simulink model "Older_model_ contains_ACC"  (R2023b)
settings: Solver=VariableStepAuto  StartTime=0.0  StopTime=30  MaxStep=1e-2  RelTol=1e-3  AbsTol=1e-3
values from neighbouring files (symbols this model uses):
  b = 1.6    [a2024_v2x_matlab_6veh.m]
  m = 2000    [a2024_v2x_matlab_6veh.m]
  mEgo = 1500    [a2024_v2x_matlab_6veh.m]
  sampleTime = 0.1    [a2024_v2x_matlab_6veh.m]    (also in v2x_matlab.m; v2x_matlabV2.m; v2x_matlab_6veh.m; v2x_matlab_R.m)
  t_gap = 1.4    [a2024_v2x_matlab_6veh.m]
  waypoints = [egoWP(:,2) egoWP(:,1), zeroforwp]    [a2024_v2x_matlab_6veh.m]    (also in misc.m = data.data.ActorSpecifications(1,1).Waypoints(:,[1,2]); v2x_matlab.m = data.data.ActorSpecifications(1,1).Waypoints(:,[1,2]); v2x_matlabV2.m = [5 -1.6 0; v2x_matlab_R.m = [5 -1.6 0)
  ZeroActors = struct(     'ActorID',0,     'Position', [1000 1000 1000],      'Velocity', [0 0 0],      'Roll', 0,      'Pitch', 0,      'Yaw', 0,      'AngularVelocity', [0 0 0])    [v2x_matlabV2.m]    (also in v2x_matlab_R.m)
undefined symbols (not defined in the file or in its folder): doppler, driving, n, PredictionHorizon, Ts
libraries: simulink x13, simulink_extras x12, commofdm x10, commdigbbndam3 x10, commchan3 x3, drivingscenarioandsensors x3, mpcadaslib x2, commsink2 x2, vehdynlibdriver x1, dspmathops x1, autolibshared x1
(part 1 of 3)
settings Model: DataDictionary=V2X.sldd  Creator=Fauszt Gábor  LastModifiedBy=Fauszt Gábor

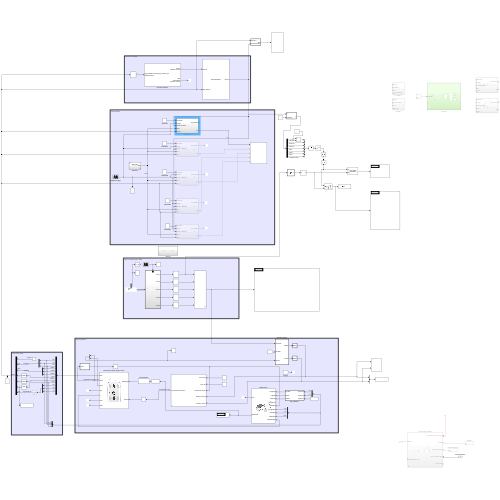
[thumbnail: Simulink's stored preview of the top-level diagram]
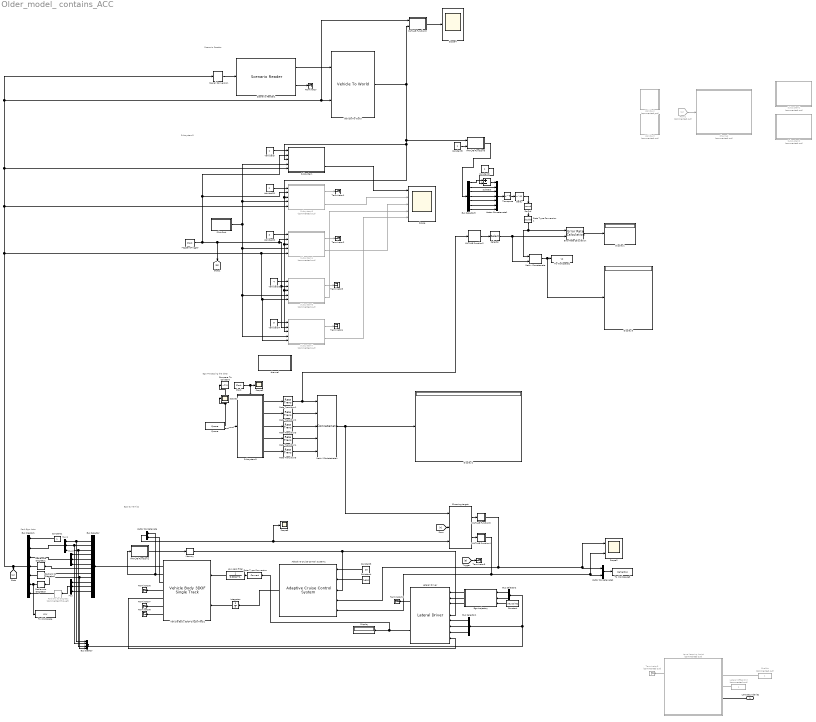
== system Older_model_ contains_ACC ==
  note: Ego Dynamics
  note: Ego Processing the data
  note: Subsystem3
  note: Scenario Reader
  note: Pack Ego Actor
  Lane Boundaries : Inport
  Adaptive Cruise Control System1 : mpcadaslib/Adaptive Cruise Control System  EgoModel=tf(1,[0.5,1,0])  InitialEgoVelocity=20  DefaultSpacing=0  MaxVelocity=20  MinAcceleration=-2  amin_ext=off  MaxAcceleration=4  amax_ext=off  Ts=0.01  PredictionHorizon=3  ControllerBehavior=0.950  suboptimal=off  maxiter=10  datatypeopt=double  optmode=off  trackmode=off
      settings: LibrarySourceBlock=mpclib/Automated Driving/Adaptive Cruise Control System
  Bus Creator : BusCreator  Inputs=4
  Bus Creator1 : BusCreator  Inputs=7  OutDataTypeStr=Bus: Actors
      settings: InheritFromInputs=off
  Bus Selector : BusSelector  OutputSignals=InertFrm.Cg.Disp.X,InertFrm.Cg.Disp.Y,InertFrm.Cg.Disp.Z,InertFrm.Cg.Vel.Xdot,InertFrm.Cg.Vel.Ydot,InertFrm.Cg.Vel.Zdot,InertFrm.Cg.Ang.phi,InertFrm.Cg.Ang.theta,InertFrm.Cg.Ang.psi,BdyFrm.Cg.AngVel.p,BdyFrm.Cg.AngVel.q,BdyFrm.Cg.AngVel.r
  Bus Selector1 : BusSelector  OutputSignals=X,Y,psi
  Bus Selector2 : BusSelector  OutputSignals=X,Y
  Bus Selector3 : BusSelector  OutputSignals=ActorID,Position,Velocity,Roll,Pitch,Yaw,AngularVelocity
  Channel : Subsystem  Commented=on
  "Choosing target " : MATLAB Function  TreatAsAtomicUnit=on
  Clock : simulink_extras/Flip Flops/Clock  period=0.01
  Compare To Constant : simulink/Logic and Bit Operations/Compare To Constant  relop=~=  const=0  OutDataTypeStr=uint8
  Constant : Constant  Value=waypoints
  Constant1 : Constant  SampleTime=-1
  Constant2 : Constant
  Constant3 : Constant  Value=20  VectorParams1D=off  SampleTime=sampleTime
  Constant4 : Constant  Value=t_gap  VectorParams1D=off  SampleTime=sampleTime
  Constant5 : Constant
  Data Type Conversion : DataTypeConversion  SaturateOnIntegerOverflow=off  RndMeth=Floor
  Data Type Conversion1 : DataTypeConversion  OutDataTypeStr=double  SaturateOnIntegerOverflow=off  RndMeth=Floor
  Delay : Delay  DelayLength=11
  Display{,1..3} (4 alike) : Display
  Ego trajectory : MATLAB Function  TreatAsAtomicUnit=on
  Enable : Constant  Commented=on
  Error Rate Calculation : commsink2/Error Rate Calculation  N=0  st_delay=0  cp_mode=Entire frame  subframe=[]  PMode=Port  WsName=ErrorVec  RsMode2=off  stop=off  numErr=100  maxBits=1e6
      settings: LibrarySourceBlock=|
      | commhdlsink/Error Rate
      | Calculation
  From : From
  From1 : From  Commented=on
  Goto : Goto
  Integrator : Integrator
  Lane Keeping Assist : Subsystem  Commented=on
  Lateral Driver : vehdynlibdriver/Lateral Driver  extSteerOvr=off  extSteerHld=off  extSteerZero=off  steerOut=off  cntrlTypeLat=Stanley  coordMode=SAE J670 (Z-down)  angUnits=rad  tau=0.1  L=3  vecPose=off  dynamMode=on  PositionGainF=2.5  PositionGainR=2.5  YawRateGain=.2  DelayGain=.2  a=a  b=b  m=mEgo  Cy_f=Cy_f  Cy_r=70933  I=4013  Ksteer=18  theta=45*pi/180  aMode=2
  Lateral Offset [m] : Constant  Commented=on
  Low pass filter : TransferFcn  Denominator=[0.001 1]
  MATLAB Function1 : MATLAB Function  TreatAsAtomicUnit=on
  MATLAB Function2 : MATLAB Function  TreatAsAtomicUnit=on
  MATLAB Function3 : MATLAB Function  TreatAsAtomicUnit=on
  MATLAB Function4 : MATLAB Function  TreatAsAtomicUnit=on
  MATLAB Function5 : MATLAB Function  TreatAsAtomicUnit=on
  MATLAB Function6 : MATLAB Function  TreatAsAtomicUnit=on
  Matrix Concatenate : Concatenate  Mode=Multidimensional array  ConcatenateDimension=2
  Matrix Concatenate1 : Concatenate  NumInputs=5  Mode=Multidimensional array  ConcatenateDimension=2
  Memory : Memory  InitialCondition=1
  MsgSendTrigger : simulink_extras/Flip Flops/Clock  period=0.1
  Mux : Mux  Inputs=3
  Mux1 : Mux  Inputs=3
  Mux2 : Mux  Inputs=3
  Pilot Port : Subsystem  ReferencedSubsystem=Pilot_Port
  Queue : Queue  OutputPortMessageModes=n,m  Capacity=5  EntityArrivalSource=Multicast  MulticastTag=B  NumberEntitiesInBlock=on
      settings: OutputPortMap=o1,o5
  Radians to Degrees : simulink_extras/Transformations/Radians to Degrees  Commented=through
  Radians to Degrees1 : simulink_extras/Transformations/Radians to Degrees
  Radians to Degrees2 : simulink_extras/Transformations/Radians to Degrees
  Radians to Degrees3 : simulink_extras/Transformations/Radians to Degrees
  Rate Transition{1..5} (5 alike) : RateTransition  OutPortSampleTime=sampleTime/10
  Round : Rounding  Operator=round
  Scenario Reader1 : drivingscenarioandsensors/Scenario Reader  ScenarioSource=From file  ScenarioFileName=C:\Users\Fauszt Gábor\OneDrive - Budapesti Műszaki és Gazdaságtudományi Egyetem\Projekt - Diplomamunka\MODELL\driving_scenario_4V.mat  ScenarioVariableName=scenario  OutputCoordinateSystem=Vehicle coordinates  EgoVehicleSource=Input port  EgoVehicleActorID=1  OrientVehiclesOnRoad=off  OutputEgoVehiclePose=on  OutputEgoVehicleState=off  SampleTime=sampleTime  LaneBoundaryOutput=All lane boundaries  LaneBoundaryDistance=0:0.5:9.5  LaneBoundaryLocation=Center of lane markings  BusNameSource=Auto  BusName=ActorsAll  BusNumActorsSource=Scenario  BusNumActors=100  BusName2Source=Auto  BusName2=BusLaneBoundaries  BusNumLaneBoundariesSource=Scenario  BusNumLaneBoundaries=10  BusName3Source=Auto  BusName3=BusEgoActor  BusName4Source=Auto  BusName4=BusEgoState  ShowCoordinateLabels=on  SimulateUsing=Interpreted execution
  Scope : Scope  NumInputPorts=5
  Scope{1,3..5} (4 alike) : Scope
  Scope2 : Scope  NumInputPorts=2
  Selector : Selector  InputPortWidth=15  IndexOptions=Starting index (dialog)  Indices=3  OutputSizes=13
  Signal Conversion : SignalConversion  ConversionOutput=Nonvirtual bus  OverrideOpt=off
  Subsystem : Subsystem
  Subsystem1 : Subsystem  Commented=on
  Subsystem2 : Subsystem  Commented=on
  Subsystem3 : Subsystem
  Subsystem4 : Subsystem  Commented=on
  Subsystem5 : Subsystem  Commented=on
  Subsystem6 : Subsystem  Commented=on
  Subsystem7 : Subsystem  Commented=on
  Subtract : Sum  Inputs=+-
  Terminator{,1..8,10} (10 alike) : Terminator
  Terminator9 : Terminator  Commented=on
  To Workspace : ToWorkspace  VariableName=yaw  SampleTime=-1
  To Workspace1 : ToWorkspace  VariableName=V2  SampleTime=-1
  To Workspace3 : ToWorkspace  VariableName=RelVelPos  SampleTime=-1
  Transpose : Math  Operator=transpose
  Vector Concatenate : Concatenate
  Vector Concatenate1 : Concatenate  NumInputs=7
  Vector Concatenate2 : Concatenate
  Vehicle 2 : Subsystem  Commented=on
  Vehicle 3 : Subsystem  Commented=on
  Vehicle Body 3DOF Single Track1 : autolibshared/Vehicle Body 3DOF Single Track  trackMode=Single (bicycle)  inputMode=External longitudinal velocity  frontSteerMode=on  rearSteerMode=off  windMode=off  muMode=off  extFMode=off  extMMode=off  htchFMode=off  htchMMode=off  extXo=off  extpsio=off  extxdoto=off  extro=off  extYo=off  extTamb=off  extydoto=off  aMode=2  NF=nrWheelsFr  NR=nrWheelsRe  m=mEgo  a=a  b=b  h=h  dh=1  hh=0.2  X_o=waypoints(1,1)  xdot_o=0  CalphaMode=off  sigmaMode=on  d=0  hl=0  w=[1.4,1.4]  Cy_f=Cy_f  Cy_r=Cy_r  sigma_f=sigma_f  sigma_r=sigma_r  alpha_f_brk=[-.1 .1]  Cy_f_data=[-9e3 9e3]  alpha_r_brk=[-.1 .1]  Cy_r_data=[-9e3 9e3]  Y_o=waypoints(1,2)  ydot_o=0  Izz=Izz  psi_o=deg2rad(waypoints(1,3))  r_o=deg2rad(waypoints(1,3))  Af=2  Cd=.3  Cl=.1  Cpm=.1  beta_w=[0 0.01:0.01:0.3]  Cs=[0 0.01:0.01:0.3]  Cym=[0 1e-6:0.01:0.3]  Pabs=101325  Tair=273  g=9.81  mu=1  xdot_tol=.01  Fznom=5000  Fxtire_sat=7e4  Fytire_sat=7e4  longOff=0  latOff=0  vertOff=0  wrapAng=off
  Vehicle To World : drivingscenarioandsensors/Vehicle To World  BusNameSource=Auto  BusName=ActorsaAll  SimulateUsing=Interpreted execution
  VehicleID : Constant
  VehicleID1 : Constant  Value=2
  VehicleID2 : Constant  Value=3
  VehicleID3 : Constant  Value=4
  VehicleID4 : Constant  Value=5
  channel : Subsystem
  wires:
  From1/1 -> Channel/1(EgoData)
  Lateral Offset [m]/1 -> Lane Keeping Assist/3(Lane Assist Offset)
  Lane Keeping Assist/1(Status) -> Terminator9/1
  Lane Boundaries/1 -> Lane Keeping Assist/4(lane boundaries Bus)
  Enable/1 -> Lane Keeping Assist/2(Enable)
  ? -> Lane Keeping Assist/1(Longitudinal velocity of ego)
  Scenario Reader1/1 -> Vehicle To World/1
  Bus Selector/6 -> Mux2/3  "<Zdot>"
  Bus Selector/5 -> Mux2/2  "<Ydot>"
  Constant1/1 -> Bus Creator1/1  "ActorID"
  Bus Selector/4 -> Mux2/1  "<Xdot>"
  Mux1/1 -> Bus Creator1/2  "Position"
  Bus Creator1/1 -> MATLAB Function3/1(EgoActor), Vehicle To World/2, Signal Conversion/1, Subsystem/5(Actors), Subsystem5/5(Actors), Subsystem7/5(Actors), Subsystem6/5(Actors), Subsystem4/5(Actors), Goto/1  "Actors"
  Bus Selector/7 -> Radians to Degrees1/1  "<phi>"
  Bus Selector/1 -> Bus Creator/1, Mux1/1  "<X>"
  Radians to Degrees/1 -> Bus Creator1/7  "AngularVelocity"
  Bus Selector/2 -> Bus Creator/2, Mux1/2  "<Y>"
  Bus Selector/10 -> Mux/1  "<p>"
  Bus Selector/8 -> Radians to Degrees2/1  "<theta>"
  Bus Selector/3 -> Mux1/3, Bus Creator/3  "<Z>"
  Mux/1 -> Radians to Degrees/1
  Mux2/1 -> Bus Creator1/3  "Velocity"
  Bus Selector/9 -> Radians to Degrees3/1, Bus Creator/4  "<psi>"
  Bus Selector/12 -> Mux/3  "<r>"
  Bus Selector/11 -> Mux/2  "<q>"
  Vehicle Body 3DOF Single Track1/1 -> Bus Selector/1
  MsgSendTrigger/1 -> Subsystem7/2(Trigger), Subsystem6/2(Trigger), Subsystem4/2(Trigger), [B], Subsystem5/2(Trigger), Subsystem/2(Trigger)
  Signal Conversion/1 -> Scenario Reader1/1
  Scenario Reader1/2 -> Terminator/1
  Radians to Degrees1/1 -> Bus Creator1/4
  Radians to Degrees2/1 -> Bus Creator1/5
  Radians to Degrees3/1 -> To Workspace/1, Bus Creator1/6
  VehicleID1/1 -> Subsystem5/1(VehicleID)
  VehicleID/1 -> Subsystem/1(VehicleID)
  Subsystem4/2(V3) -> Scope/3  "V3"
  VehicleID2/1 -> Subsystem4/1(VehicleID)
  Subsystem4/1(VehicleData) -> Terminator2/1
  Subsystem5/2(V2) -> Scope/2  "V2"
  Subsystem/2(V1) -> Scope/1  "V1"
  Vehicle To World/1 -> MATLAB Function3/2(busActors3Test1), Subsystem7/3(busActors3Test1), Subsystem6/3(busActors3Test1), Subsystem4/3(busActors3Test1), Subsystem5/3(busActors3Test1), Subsystem/3(busActors3Test1), MATLAB Function6/1(u)
  Pilot Port/1 -> Subsystem7/4(Pilot), Subsystem6/4(Pilot), Subsystem4/4(Pilot), Subsystem5/4(Pilot), Subsystem/4(Pilot)  "Pilot"
  Subsystem5/1(VehicleData) -> Terminator1/1
  [B] -> Terminator5/1
  Vector Concatenate/1 -> Scope5/1, "Choosing target "/3(EgoVel)
  Subsystem3/2(Actor2) -> Rate Transition2/1
  Matrix Concatenate1/1 -> Display2/1, "Choosing target "/1(ActorsMX)
  Subsystem3/1(Actor1) -> Rate Transition1/1
  Subsystem3/3(Actor3) -> Rate Transition3/1
  From/1 -> "Choosing target "/2(EgoData)
  Subsystem3/4(Actor4) -> Rate Transition4/1
  Queue/1 -> Compare To Constant/1, Scope1/1
  Queue/2 -> Subsystem3/1(In1)
  "Choosing target "/1(RelDist) -> MATLAB Function5/1(u)
  Bus Creator/1 -> Bus Selector2/1, Bus Selector1/1
  Memory/1 -> Lateral Driver/5, Adaptive Cruise Control System1/3
  Vehicle Body 3DOF Single Track1/2 -> Vector Concatenate/1, MATLAB Function1/1(xdotin)  "Longitudinal velocity of ego"
  Lateral Driver/1 -> Terminator10/1
  Vehicle Body 3DOF Single Track1/3 -> Vector Concatenate/2
  Data Type Conversion/1 -> Low pass filter/1
  Ego trajectory/2(LatRef) -> Lateral Driver/2
  Vehicle Body 3DOF Single Track1/5 -> Lateral Driver/9  "r"
  Bus Selector2/2 -> Ego trajectory/2(EgoFdbY)  "<Y>"
  Vehicle Body 3DOF Single Track1/6 -> Terminator7/1
  "Choosing target "/2(RelVel) -> MATLAB Function4/1(u)
  Constant/1 -> Ego trajectory/3(waypoints)
  Bus Selector1/3 -> Lateral Driver/8  "<psi>"
  Bus Selector1/1 -> Lateral Driver/6  "<X>"
  Vehicle Body 3DOF Single Track1/4 -> Terminator6/1
  Ego trajectory/1(LongRef) -> Lateral Driver/1
  Integrator/1 -> Vehicle Body 3DOF Single Track1/2
  Ego trajectory/3(YawRef) -> Lateral Driver/3
  MATLAB Function1/1(y) -> Memory/1
  Constant3/1 -> Adaptive Cruise Control System1/1
  Vehicle Body 3DOF Single Track1/7 -> Terminator8/1
  Constant4/1 -> Adaptive Cruise Control System1/2
  Low pass filter/1 -> Vehicle Body 3DOF Single Track1/1
  Bus Selector2/1 -> Ego trajectory/1(EgoFdbX)  "<X>"
  Adaptive Cruise Control System1/1 -> Integrator/1  "Acceleration of ego"
  Bus Selector1/2 -> Lateral Driver/7  "<Y>"
  Lateral Driver/2 -> Data Type Conversion/1, Display/1
  Vector Concatenate1/1 -> Transpose/1
  Bus Selector3/2 -> Vector Concatenate1/2  "<Position>"
  Bus Selector3/3 -> Vector Concatenate1/3  "<Velocity>"
  Bus Selector3/4 -> Vector Concatenate1/4  "<Roll>"
  Bus Selector3/5 -> Vector Concatenate1/5  "<Pitch>"
  Bus Selector3/6 -> Vector Concatenate1/6  "<Yaw>"
  Bus Selector3/7 -> Vector Concatenate1/7  "<AngularVelocity>"
  Selector/1 -> Matrix Concatenate/2, Error Rate Calculation/2
  Transpose/1 -> Delay/1
  MATLAB Function2/1(y) -> Selector/1
  Data Type Conversion1/1 -> Error Rate Calculation/1, Matrix Concatenate/1
  Error Rate Calculation/1 -> Display1/1
  MATLAB Function3/1(Dist) -> Scope4/1
  Matrix Concatenate/1 -> Display3/1, To Workspace1/1
  Round/1 -> Data Type Conversion1/1
  Vector Concatenate2/1 -> To Workspace3/1
  MATLAB Function4/1(RelVel) -> Adaptive Cruise Control System1/5, Scope2/2, Vector Concatenate2/2
  MATLAB Function5/1(RelDist) -> Adaptive Cruise Control System1/4, Vector Concatenate2/1, Scope2/1
  Delay/1 -> Round/1
  Clock/1 -> Scope3/1, Subsystem3/Enable
  Rate Transition3/1 -> Matrix Concatenate1/3
  Rate Transition2/1 -> Matrix Concatenate1/2
  Rate Transition1/1 -> MATLAB Function2/1(u), Matrix Concatenate1/1
  Rate Transition4/1 -> Matrix Concatenate1/4
  MATLAB Function6/1(y) -> Bus Selector3/1
  VehicleID3/1 -> Subsystem6/1(VehicleID)
  VehicleID4/1 -> Subsystem7/1(VehicleID)
  Subsystem6/1(VehicleData) -> Terminator3/1
  Subsystem7/1(VehicleData) -> Terminator4/1
  Subsystem3/5(Actor5) -> Rate Transition5/1
  Rate Transition5/1 -> Matrix Concatenate1/5
  Subsystem6/2(V4) -> Scope/4  "V4"
  Subsystem7/2(V5) -> Scope/5  "V3"
  Bus Selector3/1 -> Subtract/1  "<ActorID>"
  Subtract/1 -> Vector Concatenate1/1
  Constant2/1 -> Subtract/2
  Constant5/1 -> MATLAB Function6/2(vehicleID)

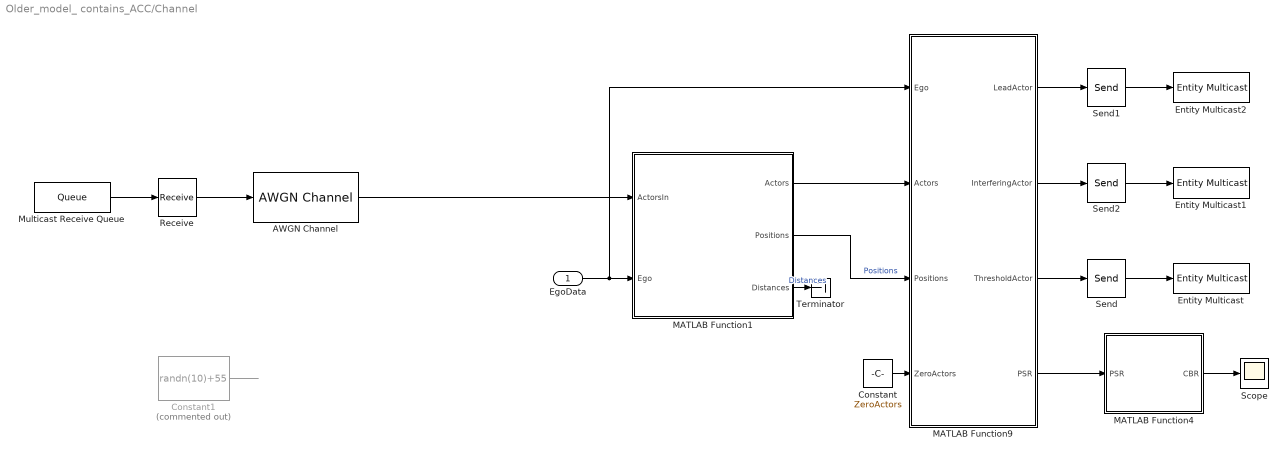
== system Older_model_ contains_ACC/Channel ==
  EgoData : Inport
  AWGN Channel : commchan3/AWGN Channel  LegacyMode=off  NoiseMethod="Signal to noise ratio  (SNR)"  noiseMode="Signal to noise ratio  (SNR)"  EbNo=10  EsNo=10  SNR=60  BitsPerSymbol=1  SignalPower=1  SamplesPerSymbol=1  SymbolPeriod=1  VarianceSource=Parameter  Variance=1  RandomStream=Global stream  Seed=67  SimulateUsing=Interpreted execution
  Constant : Constant  Value=ZeroActors  OutDataTypeStr=Bus: Actors  SampleTime=sampleTime
  Constant1 : Constant  Commented=on  Value=randn(10)+55  SampleTime=sampleTime
  Entity Multicast : EntityMulticast  InputPortMessageModes=m  MulticastTag=B
  Entity Multicast1 : EntityMulticast  InputPortMessageModes=m  MulticastTag=B
  Entity Multicast2 : EntityMulticast  InputPortMessageModes=m  MulticastTag=B
  MATLAB Function1 : MATLAB Function  TreatAsAtomicUnit=on
  MATLAB Function4 : MATLAB Function  TreatAsAtomicUnit=on
  MATLAB Function9 : MATLAB Function  TreatAsAtomicUnit=on
  Multicast Receive Queue : Queue  OutputPortMessageModes=m  EntityArrivalSource=Multicast
  Receive : Receive  InputPortMessageModes=m  UseInternalQueue=off  QueueOverwriting=on  QueueLength=1  QueueType=LIFO
  Scope : Scope
  Send : Send  OutputPortMessageModes=m
  Send1 : Send  OutputPortMessageModes=m
  Send2 : Send  OutputPortMessageModes=m
  Terminator : Terminator
  wires:
  Multicast Receive Queue/1 -> Receive/1
  AWGN Channel/1 -> MATLAB Function1/1(ActorsIn)
  Receive/1 -> AWGN Channel/1
  MATLAB Function1/1(Actors) -> MATLAB Function9/2(Actors)
  MATLAB Function1/2(Positions) -> MATLAB Function9/3(Positions)  "Positions"
  Constant/1 -> MATLAB Function9/4(ZeroActors)
  MATLAB Function9/4(PSR) -> MATLAB Function4/1(PSR)
  MATLAB Function9/3(ThresholdActor) -> Send/1
  MATLAB Function9/2(InterferingActor) -> Send2/1
  MATLAB Function9/1(LeadActor) -> Send1/1
  EgoData/1 -> MATLAB Function9/1(Ego), MATLAB Function1/2(Ego)
  Constant1/1 -> ?
  MATLAB Function1/3(Distances) -> Terminator/1  "Distances"
  MATLAB Function4/1(CBR) -> Scope/1
  Send1/1 -> Entity Multicast2/1
  Send2/1 -> Entity Multicast1/1
  Send/1 -> Entity Multicast/1

== system Older_model_ contains_ACC/Lane Keeping Assist ==
  Longitudinal velocity of ego : Inport
  Enable : Inport  Port=2
  Lane Assist Offset : Inport  Port=3
  lane boundaries Bus : Inport  Port=4
  Driver Steer : Inport  Port=5
  Abs : Abs  SaturateOnIntegerOverflow=off
  Estimate lane center : Subsystem
  Lane Keeping Assist System : mpcadaslib/Lane Keeping Assist System  ModelType=Use vehicle parameters  VehicleMass=mEgo  VehicleYawInertia=2875  LengthToFront=a  LengthToRear=b  FrontTireStiffness=Cy_f  RearTireStiffness=Cy_r  EgoModelMatrixA=[-4.4021 ,-12.4603;1.3913,-5.1868]  EgoModelMatrixB=[24.1270;15.8609]  EgoModelMatrixC=[1,0;0,1]  InitialLongVel=16  TransportLag=0  MinSteering=-0.5  umin_ext=off  MaxSteering=0.5  umax_ext=off  Ts=0.1  PredictionHorizon=5  ControllerBehavior=0.100  suboptimal=off  maxiter=10  datatypeopt=double  optmode=off  trackmode=off
      link override Longitudinal velocity must be positive: stopWhenAssertionFail=on
      settings: LibrarySourceBlock=mpclib/Automated Driving/Lane Keeping Assist System
  Pack to Custom Sensor Data Format : Subsystem
  Subsystem : Subsystem
  Subsystem2 : Subsystem
  Vision Detection Generator : drivingscenarioandsensors/Vision Detection Generator  SensorIndex=1  DetectorOutput=Lanes only  UpdateInterval=0.1  LaneUpdateInterval=0.1  SensorLocation=[ 1.9, 0 ]  Height=1.1  Yaw=0  Pitch=1  Roll=0  BusNameSource=Auto  BusName=BusObjectDetections  BusName2Source=Auto  BusName2=BusLaneDetections  MaxNumDetectionsSource=Property  MaxNumDetections=50  MaxNumLanesSource=Property  MaxNumLanes=30  DetectionCoordinates=Ego Cartesian  SimulateUsing=Interpreted execution  MaxRange=10  BoundingBoxAccuracy=5  ProcessNoiseIntensity=5  MaxSpeed=100  MaxAllowedOcclusion=0.5  MinObjectImageSize=[ 15, 15 ]  DetectionProbability=0.9  FalsePositivesPerImage=0.1  MinLaneImageSize=[ 20, 3 ]  LaneBoundaryAccuracy=3  HasNoise=on  InitialSeedSource=Repeatable  InitialSeed=0  UsedSeed=driving.internal.SimulinkUtilities.seedManager(gcb)  ActorProfilesSource=From Scenario Reader block  ActorProfilesParameters=driving.internal.ActorProfilesParameters  ActorProfilesExpression=struct( 'ClassID', 0, 'Length', 4.7, 'Width', 1.8, 'Height', 1.4, 'OriginOffset', [ -1.35, 0, 0 ] )  Intrinsics=driving.internal.cameraIntrinsics('FocalLength',[1, 1 ])
  Status : Outport
  SteeringAngle in rad : Outport  Port=2
  wires:
  Subsystem/1(Departure Detected) -> Subsystem2/2(Set)
  Estimate lane center/2(Lateral Offset) -> Lane Keeping Assist System/3
  Enable/1 -> Subsystem2/1(Enable)
  Pack to Custom Sensor Data Format/1(lanes) -> Subsystem/2(Lane Sensor data), Estimate lane center/2(Lane Boundaries)
  Estimate lane center/1(Previewed Curvature) -> Lane Keeping Assist System/1
  Estimate lane center/3(Heading Angle) -> Lane Keeping Assist System/4
  lane boundaries Bus/1 -> Vision Detection Generator/1
  Vision Detection Generator/1 -> Pack to Custom Sensor Data Format/1(lane Detections)
  Lane Assist Offset/1 -> Subsystem/1(Lane Assist Offset)
  Driver Steer/1 -> Subsystem2/4(Driver Steer)
  Subsystem2/1(Status) -> Status/1
  Longitudinal velocity of ego/1 -> Abs/1, Estimate lane center/1(Longitudinal velocity of ego)
  Abs/1 -> Lane Keeping Assist System/2
  Subsystem2/2(SteeringAngle in rad) -> SteeringAngle in rad/1
  Lane Keeping Assist System/1 -> Subsystem2/3(Assisted Steer)  "Assisted Steer"

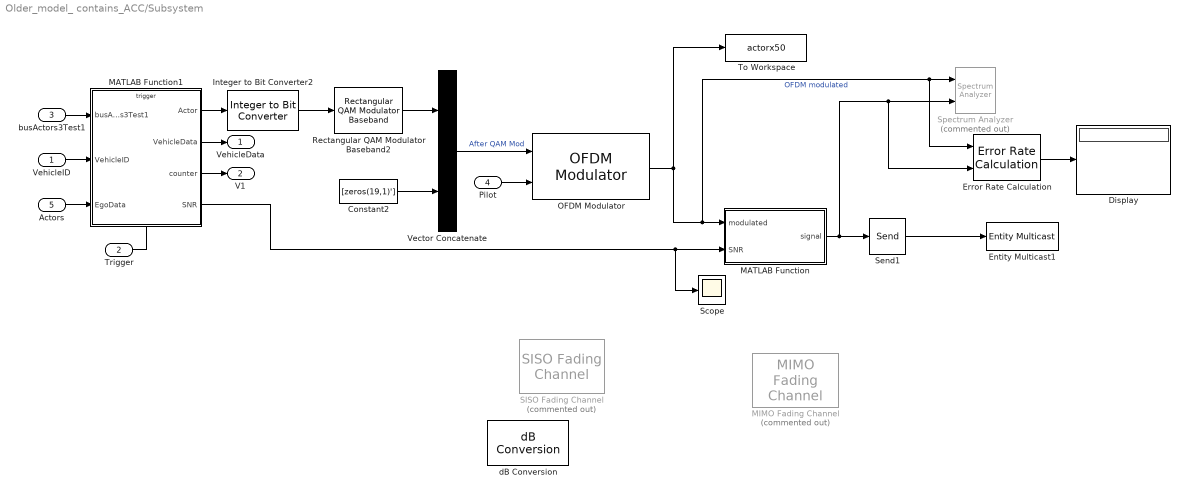
== system Older_model_ contains_ACC/Subsystem ==
  VehicleID : Inport
  Trigger : Inport  Port=2
  busActors3Test1 : Inport  Port=3
  Pilot : Inport  Port=4
  Actors : Inport  Port=5
  Constant2 : Constant  Value=[zeros(19,1)']  SampleTime=-1
  Display : Display
  Entity Multicast1 : EntityMulticast  InputPortMessageModes=m
  Error Rate Calculation : commsink2/Error Rate Calculation  N=0  st_delay=0  cp_mode=Entire frame  subframe=[]  PMode=Port  WsName=ErrorVec  RsMode2=off  stop=off  numErr=100  maxBits=1e6
      settings: LibrarySourceBlock=|
      | commhdlsink/Error Rate
      | Calculation
  Integer to Bit Converter2 : simulink/Logic and Bit Operations/Integer to Bit Converter  nbits=16  signedInputValues=Signed  bitOrder=MSB first  outDtype=boolean
  MATLAB Function : MATLAB Function  TreatAsAtomicUnit=on
  MATLAB Function1 : MATLAB Function  TreatAsAtomicUnit=on
  MIMO Fading Channel : commchan3/MIMO Fading Channel  Commented=on  InheritSampleRate=on  SampleRate=1  PathDelays=0  AveragePathGains=0  NormalizePathGains=on  FadingDistribution=Rayleigh  KFactor=3  DirectPathDopplerShift=0  DirectPathInitialPhase=0  MaximumDopplerShift=0.001  DopplerSpectrum=doppler('Jakes')  SpatialCorrelationSpecification=None  SpatialCorrelationMatrix=[1 0 0 0; 0 1 0 0; 0 0 1 0; 0 0 0 1]  NumTransmitAntennas=1  NumReceiveAntennas=1  TransmitCorrelationMatrix=[1 0; 0 1]  ReceiveCorrelationMatrix=[1 0; 0 1]  AntennaSelection=Off  NormalizeChannelOutputs=on  PathGainsOutputPort=off  SimulateUsing=Interpreted execution  FadingTechnique=Filtered Gaussian noise  NumSinusoids=48  InitialTimeSource=Property  InitialTime=0  RandomStream=mt19937ar with seed  Seed=73  Visualization=Off  AntennaPairsToDisplay=[ 1, 1 ]  PathsForDopplerDisplay=1  SamplesToDisplay=25%
  OFDM Modulator : commofdm/OFDM Modulator  StatePerturbationForJacobian=1.0e-05  FFTLength=64  NumGuardBandCarriers=[0;0]  InsertDCNull=on  PilotInputPort=on  PilotCarrierIndices=[12; 26; 40; 54]  CyclicPrefixLength=32  Windowing=off  WindowLength=16  OversamplingFactor=3  NumSymbols=1  NumTransmitAntennas=1  SimulateUsing=Interpreted execution
  Rectangular QAM Modulator Baseband2 : commdigbbndam3/Rectangular QAM Modulator Baseband  M=2^6  InType=Bit  Enc=Binary  Mapping=[0:15]  PowType=Average Power  MinDist=2  AvgPow=P_Signal  PeakPow=1  Ph=0  outDtype=double  outWordLen=16  outUDDataType=sfix(16)  outFracLenMode=Best precision  outFracLen=15  outDataTypeStr=double  outLastDataTypeStr=double
      settings: LibrarySourceBlock=|
      | commhdldigbbndam/Rectangular QAM
      | Modulator
      | Baseband
  SISO Fading Channel : commchan3/SISO Fading Channel  Commented=on  InheritSampleRate=off  SampleRate=5.9e9  PathDelays=0  AveragePathGains=0  NormalizePathGains=on  FadingDistribution=Rayleigh  KFactor=3  DirectPathDopplerShift=0  DirectPathInitialPhase=0  MaximumDopplerShift=0.001  DopplerSpectrum=doppler('Jakes')  RandomStream=mt19937ar with seed  Seed=73  PathGainsOutputPort=off  ChannelFilterDelayOutputPort=off  SimulateUsing=Interpreted execution  Visualization=Off  PathsForDopplerDisplay=1  SamplesToDisplay=25%
  Scope : Scope
  Send1 : Send  OutputPortMessageModes=m
  Spectrum Analyzer : SpectrumAnalyzer  Commented=on  NumInputPorts=2  WindowPosition=[448.000000,229.000000,892.000000,599.000000,]  ScopeFrameLocation=window  Span=28800  StartFrequency=-14400  StopFrequency=14400  YLimits=[-76.87471744,11.31414123]  ColorLimits=[-74.70368596,10.48749861]  ShowLegend=on
  To Workspace : ToWorkspace  VariableName=actorx50  SampleTime=-1
  Vector Concatenate : Concatenate
  dB Conversion : dspmathops/dB Conversion  dBtype=dB  intype=Amplitude  R=1  fuzz=off
      settings: LibrarySourceBlock=commutil2/dB Conversion
  VehicleData : Outport
  V1 : Outport  Port=2
  wires:
  MATLAB Function1/1(Actor) -> Integer to Bit Converter2/1
  Vector Concatenate/1 -> OFDM Modulator/1  "After QAM Mod"
  Send1/1 -> Entity Multicast1/1
  Rectangular QAM Modulator Baseband2/1 -> Vector Concatenate/1
  Constant2/1 -> Vector Concatenate/2
  Actors/1 -> MATLAB Function1/3(EgoData)
  OFDM Modulator/1 -> MATLAB Function/1(modulated), Error Rate Calculation/1, Spectrum Analyzer/1, To Workspace/1  "OFDM modulated"
  Integer to Bit Converter2/1 -> Rectangular QAM Modulator Baseband2/1
  busActors3Test1/1 -> MATLAB Function1/1(busActors3Test1)
  VehicleID/1 -> MATLAB Function1/2(VehicleID)
  Pilot/1 -> OFDM Modulator/2
  MATLAB Function1/2(VehicleData) -> VehicleData/1
  MATLAB Function1/3(counter) -> V1/1
  Trigger/1 -> MATLAB Function1/Trigger
  Error Rate Calculation/1 -> Display/1
  MATLAB Function/1(signal) -> Error Rate Calculation/2, Spectrum Analyzer/2, Send1/1
  MATLAB Function1/4(SNR) -> Scope/1, MATLAB Function/2(SNR)

== system Older_model_ contains_ACC/Subsystem1 ==
  VehicleID : Inport
  Trigger : Inport  Port=2
  busActors3Test1 : Inport  Port=3
  Pilot : Inport  Port=4
  Actors : Inport  Port=5
  Constant2 : Constant  Value=[zeros(19,1)']  SampleTime=-1
  Entity Multicast1 : EntityMulticast  InputPortMessageModes=m
  Integer to Bit Converter2 : simulink/Logic and Bit Operations/Integer to Bit Converter  nbits=16  signedInputValues=Signed  bitOrder=MSB first  outDtype=boolean
  MATLAB Function1 : MATLAB Function  TreatAsAtomicUnit=on
  OFDM Modulator : commofdm/OFDM Modulator  StatePerturbationForJacobian=1.0e-05  FFTLength=64  NumGuardBandCarriers=[0;0]  InsertDCNull=on  PilotInputPort=on  PilotCarrierIndices=[12; 26; 40; 54]  CyclicPrefixLength=32  Windowing=off  WindowLength=16  OversamplingFactor=3  NumSymbols=1  NumTransmitAntennas=1  SimulateUsing=Interpreted execution
  Rectangular QAM Modulator Baseband2 : commdigbbndam3/Rectangular QAM Modulator Baseband  M=2^6  InType=Bit  Enc=Binary  Mapping=[0:15]  PowType=Average Power  MinDist=2  AvgPow=P_Signal  PeakPow=1  Ph=0  outDtype=double  outWordLen=16  outUDDataType=sfix(16)  outFracLenMode=Best precision  outFracLen=15  outDataTypeStr=double  outLastDataTypeStr=double
      settings: LibrarySourceBlock=|
      | commhdldigbbndam/Rectangular QAM
      | Modulator
      | Baseband
  Send1 : Send  OutputPortMessageModes=m
  Vector Concatenate : Concatenate
  VehicleData : Outport
  V2 : Outport  Port=2
  wires:
  MATLAB Function1/3(counter) -> V2/1
  MATLAB Function1/2(VehicleData) -> VehicleData/1
  Pilot/1 -> OFDM Modulator/2
  VehicleID/1 -> MATLAB Function1/2(VehicleID)
  busActors3Test1/1 -> MATLAB Function1/1(busActors3Test1)
  Trigger/1 -> MATLAB Function1/Trigger
  Integer to Bit Converter2/1 -> Rectangular QAM Modulator Baseband2/1
  OFDM Modulator/1 -> Send1/1  "OFDM modulated"
  Actors/1 -> MATLAB Function1/3(EgoData)
  Constant2/1 -> Vector Concatenate/2
  Rectangular QAM Modulator Baseband2/1 -> Vector Concatenate/1
  Send1/1 -> Entity Multicast1/1
  Vector Concatenate/1 -> OFDM Modulator/1  "After QAM Mod"
  MATLAB Function1/1(Actor) -> Integer to Bit Converter2/1

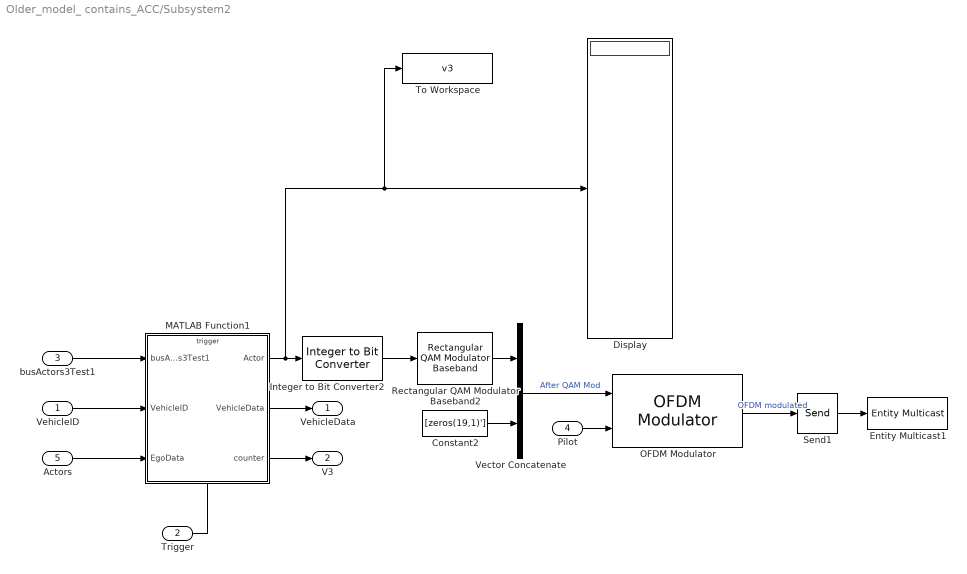
== system Older_model_ contains_ACC/Subsystem2 ==
  VehicleID : Inport
  Trigger : Inport  Port=2
  busActors3Test1 : Inport  Port=3
  Pilot : Inport  Port=4
  Actors : Inport  Port=5
  Constant2 : Constant  Value=[zeros(19,1)']  SampleTime=-1
  Display : Display
  Entity Multicast1 : EntityMulticast  InputPortMessageModes=m
  Integer to Bit Converter2 : simulink/Logic and Bit Operations/Integer to Bit Converter  nbits=16  signedInputValues=Signed  bitOrder=MSB first  outDtype=boolean
  MATLAB Function1 : MATLAB Function  TreatAsAtomicUnit=on
  OFDM Modulator : commofdm/OFDM Modulator  StatePerturbationForJacobian=1.0e-05  FFTLength=64  NumGuardBandCarriers=[0;0]  InsertDCNull=on  PilotInputPort=on  PilotCarrierIndices=[12; 26; 40; 54]  CyclicPrefixLength=32  Windowing=off  WindowLength=16  OversamplingFactor=3  NumSymbols=1  NumTransmitAntennas=1  SimulateUsing=Interpreted execution
  Rectangular QAM Modulator Baseband2 : commdigbbndam3/Rectangular QAM Modulator Baseband  M=2^6  InType=Bit  Enc=Binary  Mapping=[0:15]  PowType=Average Power  MinDist=2  AvgPow=P_Signal  PeakPow=1  Ph=0  outDtype=double  outWordLen=16  outUDDataType=sfix(16)  outFracLenMode=Best precision  outFracLen=15  outDataTypeStr=double  outLastDataTypeStr=double
      settings: LibrarySourceBlock=|
      | commhdldigbbndam/Rectangular QAM
      | Modulator
      | Baseband
  Send1 : Send  OutputPortMessageModes=m
  To Workspace : ToWorkspace  VariableName=v3  SampleTime=-1
  Vector Concatenate : Concatenate
  VehicleData : Outport
  V3 : Outport  Port=2
  wires:
  MATLAB Function1/1(Actor) -> To Workspace/1, Display/1, Integer to Bit Converter2/1
  Vector Concatenate/1 -> OFDM Modulator/1  "After QAM Mod"
  Send1/1 -> Entity Multicast1/1
  Rectangular QAM Modulator Baseband2/1 -> Vector Concatenate/1
  Constant2/1 -> Vector Concatenate/2
  Actors/1 -> MATLAB Function1/3(EgoData)
  OFDM Modulator/1 -> Send1/1  "OFDM modulated"
  Integer to Bit Converter2/1 -> Rectangular QAM Modulator Baseband2/1
  Trigger/1 -> MATLAB Function1/Trigger
  busActors3Test1/1 -> MATLAB Function1/1(busActors3Test1)
  VehicleID/1 -> MATLAB Function1/2(VehicleID)
  Pilot/1 -> OFDM Modulator/2
  MATLAB Function1/2(VehicleData) -> VehicleData/1
  MATLAB Function1/3(counter) -> V3/1

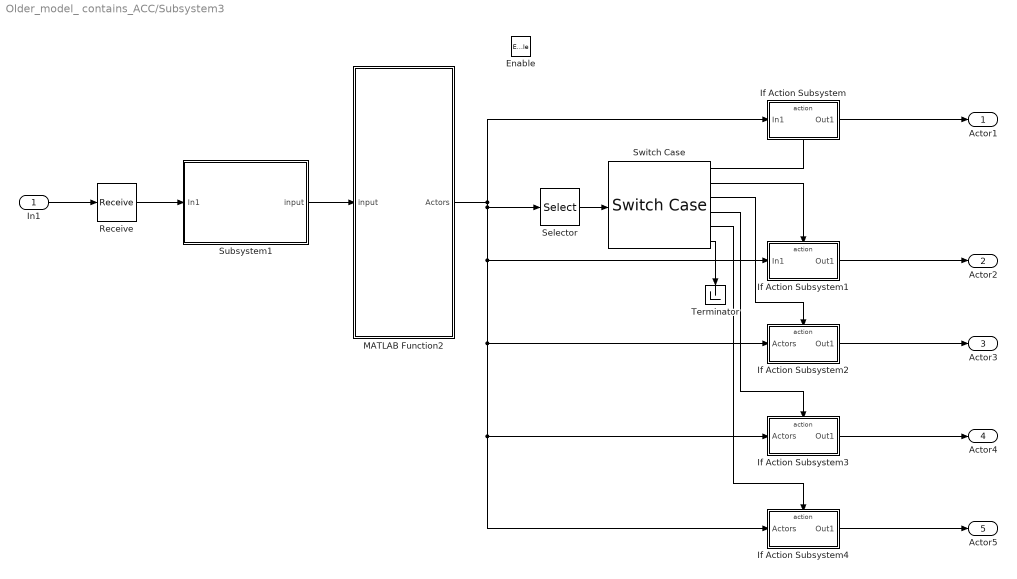
== system Older_model_ contains_ACC/Subsystem3 ==
  In1 : Inport
  Enable : EnablePort
  If Action Subsystem : Subsystem  TreatAsAtomicUnit=on
  If Action Subsystem1 : Subsystem  TreatAsAtomicUnit=on
  If Action Subsystem2 : Subsystem  TreatAsAtomicUnit=on
  If Action Subsystem3 : Subsystem  TreatAsAtomicUnit=on
  If Action Subsystem4 : Subsystem  TreatAsAtomicUnit=on
  MATLAB Function2 : MATLAB Function  TreatAsAtomicUnit=on  SystemSampleTime=0.01
  Receive : Receive  InputPortMessageModes=m  UseInternalQueue=off  QueueOverwriting=on  QueueLength=1  QueueType=LIFO
  Selector : Selector  InputPortWidth=15  IndexOptions=Index vector (dialog)  Indices=[3]  OutputSizes=1
  Subsystem1 : Subsystem
  Switch Case : SwitchCase  CaseConditions={1,2,3,4,5}
  Terminator : Terminator
  Actor1 : Outport
  Actor2 : Outport  Port=2
  Actor3 : Outport  Port=3
  Actor4 : Outport  Port=4
  Actor5 : Outport  Port=5
  wires:
  Selector/1 -> Switch Case/1
  Switch Case/1 -> If Action Subsystem/Action
  If Action Subsystem/1(Out1) -> Actor1/1
  If Action Subsystem1/1(Out1) -> Actor2/1
  Switch Case/2 -> If Action Subsystem1/Action
  Receive/1 -> Subsystem1/1(In1)
  In1/1 -> Receive/1
  Subsystem1/1(input) -> MATLAB Function2/1(input)
  If Action Subsystem2/1(Out1) -> Actor3/1
  Switch Case/3 -> If Action Subsystem2/Action
  If Action Subsystem3/1(Out1) -> Actor4/1
  MATLAB Function2/1(Actors) -> Selector/1, If Action Subsystem4/1(Actors), If Action Subsystem3/1(Actors), If Action Subsystem2/1(Actors), If Action Subsystem1/1(In1), If Action Subsystem/1(In1)
  Switch Case/4 -> If Action Subsystem3/Action
  Switch Case/6 -> Terminator/1
  If Action Subsystem4/1(Out1) -> Actor5/1
  Switch Case/5 -> If Action Subsystem4/Action

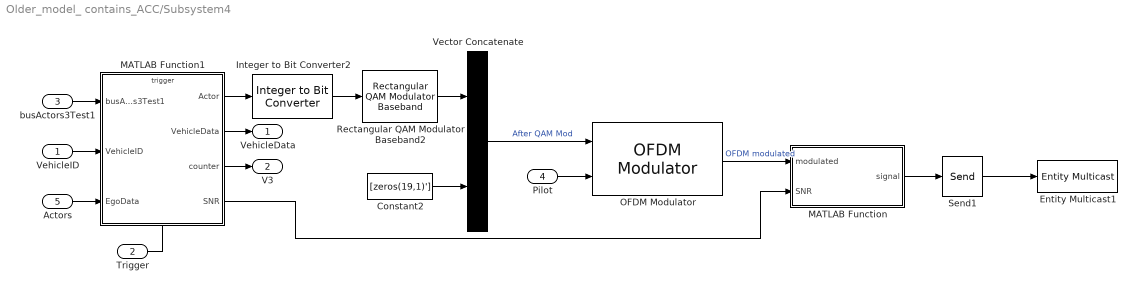
== system Older_model_ contains_ACC/Subsystem4 ==
  VehicleID : Inport
  Trigger : Inport  Port=2
  busActors3Test1 : Inport  Port=3
  Pilot : Inport  Port=4
  Actors : Inport  Port=5
  Constant2 : Constant  Value=[zeros(19,1)']  SampleTime=-1
  Entity Multicast1 : EntityMulticast  InputPortMessageModes=m
  Integer to Bit Converter2 : simulink/Logic and Bit Operations/Integer to Bit Converter  nbits=16  signedInputValues=Signed  bitOrder=MSB first  outDtype=boolean
  MATLAB Function : MATLAB Function  TreatAsAtomicUnit=on
  MATLAB Function1 : MATLAB Function  TreatAsAtomicUnit=on
  OFDM Modulator : commofdm/OFDM Modulator  StatePerturbationForJacobian=1.0e-05  FFTLength=64  NumGuardBandCarriers=[0;0]  InsertDCNull=on  PilotInputPort=on  PilotCarrierIndices=[12; 26; 40; 54]  CyclicPrefixLength=32  Windowing=off  WindowLength=16  OversamplingFactor=3  NumSymbols=1  NumTransmitAntennas=1  SimulateUsing=Interpreted execution
  Rectangular QAM Modulator Baseband2 : commdigbbndam3/Rectangular QAM Modulator Baseband  M=2^6  InType=Bit  Enc=Binary  Mapping=[0:15]  PowType=Average Power  MinDist=2  AvgPow=P_Signal  PeakPow=1  Ph=0  outDtype=double  outWordLen=16  outUDDataType=sfix(16)  outFracLenMode=Best precision  outFracLen=15  outDataTypeStr=double  outLastDataTypeStr=double
      settings: LibrarySourceBlock=|
      | commhdldigbbndam/Rectangular QAM
      | Modulator
      | Baseband
  Send1 : Send  OutputPortMessageModes=m
  Vector Concatenate : Concatenate
  VehicleData : Outport
  V3 : Outport  Port=2
  wires:
  MATLAB Function1/4(SNR) -> MATLAB Function/2(SNR)
  MATLAB Function1/3(counter) -> V3/1
  MATLAB Function1/2(VehicleData) -> VehicleData/1
  Pilot/1 -> OFDM Modulator/2
  VehicleID/1 -> MATLAB Function1/2(VehicleID)
  busActors3Test1/1 -> MATLAB Function1/1(busActors3Test1)
  Integer to Bit Converter2/1 -> Rectangular QAM Modulator Baseband2/1
  OFDM Modulator/1 -> MATLAB Function/1(modulated)  "OFDM modulated"
  Actors/1 -> MATLAB Function1/3(EgoData)
  Constant2/1 -> Vector Concatenate/2
  Rectangular QAM Modulator Baseband2/1 -> Vector Concatenate/1
  Send1/1 -> Entity Multicast1/1
  Vector Concatenate/1 -> OFDM Modulator/1  "After QAM Mod"
  MATLAB Function1/1(Actor) -> Integer to Bit Converter2/1
  Trigger/1 -> MATLAB Function1/Trigger
  MATLAB Function/1(signal) -> Send1/1

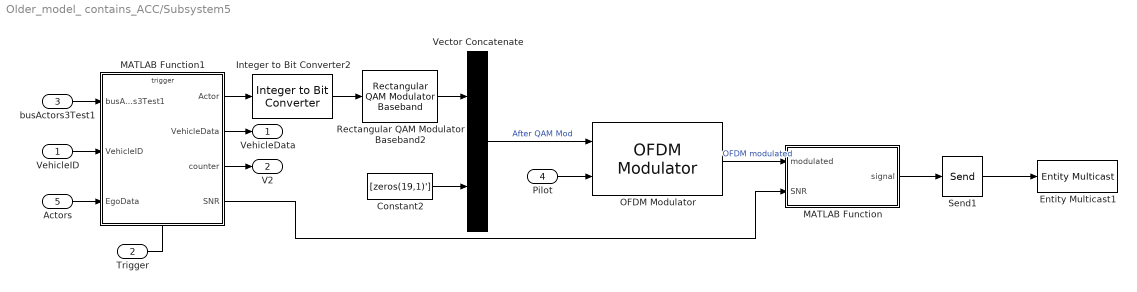
== system Older_model_ contains_ACC/Subsystem5 ==
  VehicleID : Inport
  Trigger : Inport  Port=2
  busActors3Test1 : Inport  Port=3
  Pilot : Inport  Port=4
  Actors : Inport  Port=5
  Constant2 : Constant  Value=[zeros(19,1)']  SampleTime=-1
  Entity Multicast1 : EntityMulticast  InputPortMessageModes=m
  Integer to Bit Converter2 : simulink/Logic and Bit Operations/Integer to Bit Converter  nbits=16  signedInputValues=Signed  bitOrder=MSB first  outDtype=boolean
  MATLAB Function : MATLAB Function  TreatAsAtomicUnit=on
  MATLAB Function1 : MATLAB Function  TreatAsAtomicUnit=on
  OFDM Modulator : commofdm/OFDM Modulator  StatePerturbationForJacobian=1.0e-05  FFTLength=64  NumGuardBandCarriers=[0;0]  InsertDCNull=on  PilotInputPort=on  PilotCarrierIndices=[12; 26; 40; 54]  CyclicPrefixLength=32  Windowing=off  WindowLength=16  OversamplingFactor=3  NumSymbols=1  NumTransmitAntennas=1  SimulateUsing=Interpreted execution
  Rectangular QAM Modulator Baseband2 : commdigbbndam3/Rectangular QAM Modulator Baseband  M=2^6  InType=Bit  Enc=Binary  Mapping=[0:15]  PowType=Average Power  MinDist=2  AvgPow=P_Signal  PeakPow=1  Ph=0  outDtype=double  outWordLen=16  outUDDataType=sfix(16)  outFracLenMode=Best precision  outFracLen=15  outDataTypeStr=double  outLastDataTypeStr=double
      settings: LibrarySourceBlock=|
      | commhdldigbbndam/Rectangular QAM
      | Modulator
      | Baseband
  Send1 : Send  OutputPortMessageModes=m
  Vector Concatenate : Concatenate
  VehicleData : Outport
  V2 : Outport  Port=2
  wires:
  MATLAB Function1/4(SNR) -> MATLAB Function/2(SNR)
  MATLAB Function/1(signal) -> Send1/1
  MATLAB Function1/3(counter) -> V2/1
  MATLAB Function1/2(VehicleData) -> VehicleData/1
  Pilot/1 -> OFDM Modulator/2
  VehicleID/1 -> MATLAB Function1/2(VehicleID)
  busActors3Test1/1 -> MATLAB Function1/1(busActors3Test1)
  Trigger/1 -> MATLAB Function1/Trigger
  Integer to Bit Converter2/1 -> Rectangular QAM Modulator Baseband2/1
  OFDM Modulator/1 -> MATLAB Function/1(modulated)  "OFDM modulated"
  Actors/1 -> MATLAB Function1/3(EgoData)
  Constant2/1 -> Vector Concatenate/2
  Rectangular QAM Modulator Baseband2/1 -> Vector Concatenate/1
  Send1/1 -> Entity Multicast1/1
  Vector Concatenate/1 -> OFDM Modulator/1  "After QAM Mod"
  MATLAB Function1/1(Actor) -> Integer to Bit Converter2/1

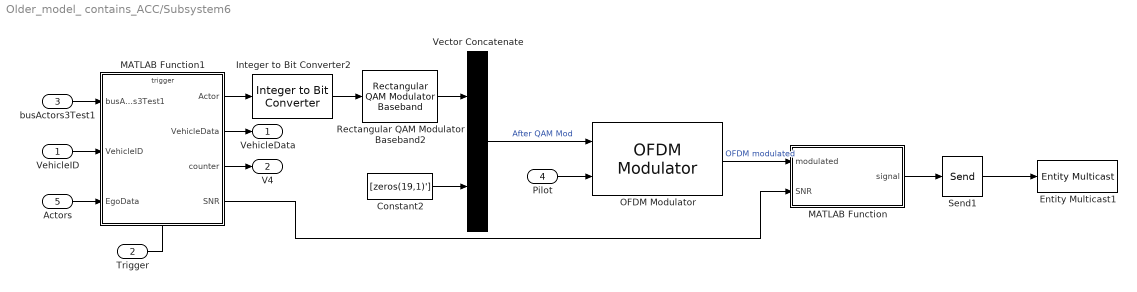
== system Older_model_ contains_ACC/Subsystem6 ==
  VehicleID : Inport
  Trigger : Inport  Port=2
  busActors3Test1 : Inport  Port=3
  Pilot : Inport  Port=4
  Actors : Inport  Port=5
  Constant2 : Constant  Value=[zeros(19,1)']  SampleTime=-1
  Entity Multicast1 : EntityMulticast  InputPortMessageModes=m
  Integer to Bit Converter2 : simulink/Logic and Bit Operations/Integer to Bit Converter  nbits=16  signedInputValues=Signed  bitOrder=MSB first  outDtype=boolean
  MATLAB Function : MATLAB Function  TreatAsAtomicUnit=on
  MATLAB Function1 : MATLAB Function  TreatAsAtomicUnit=on
  OFDM Modulator : commofdm/OFDM Modulator  StatePerturbationForJacobian=1.0e-05  FFTLength=64  NumGuardBandCarriers=[0;0]  InsertDCNull=on  PilotInputPort=on  PilotCarrierIndices=[12; 26; 40; 54]  CyclicPrefixLength=32  Windowing=off  WindowLength=16  OversamplingFactor=3  NumSymbols=1  NumTransmitAntennas=1  SimulateUsing=Interpreted execution
  Rectangular QAM Modulator Baseband2 : commdigbbndam3/Rectangular QAM Modulator Baseband  M=2^6  InType=Bit  Enc=Binary  Mapping=[0:15]  PowType=Average Power  MinDist=2  AvgPow=P_Signal  PeakPow=1  Ph=0  outDtype=double  outWordLen=16  outUDDataType=sfix(16)  outFracLenMode=Best precision  outFracLen=15  outDataTypeStr=double  outLastDataTypeStr=double
      settings: LibrarySourceBlock=|
      | commhdldigbbndam/Rectangular QAM
      | Modulator
      | Baseband
  Send1 : Send  OutputPortMessageModes=m
  Vector Concatenate : Concatenate
  VehicleData : Outport
  V4 : Outport  Port=2
  wires:
  MATLAB Function1/4(SNR) -> MATLAB Function/2(SNR)
  MATLAB Function1/3(counter) -> V4/1
  MATLAB Function1/2(VehicleData) -> VehicleData/1
  Pilot/1 -> OFDM Modulator/2
  VehicleID/1 -> MATLAB Function1/2(VehicleID)
  busActors3Test1/1 -> MATLAB Function1/1(busActors3Test1)
  Integer to Bit Converter2/1 -> Rectangular QAM Modulator Baseband2/1
  OFDM Modulator/1 -> MATLAB Function/1(modulated)  "OFDM modulated"
  Actors/1 -> MATLAB Function1/3(EgoData)
  Constant2/1 -> Vector Concatenate/2
  Rectangular QAM Modulator Baseband2/1 -> Vector Concatenate/1
  Send1/1 -> Entity Multicast1/1
  Vector Concatenate/1 -> OFDM Modulator/1  "After QAM Mod"
  MATLAB Function1/1(Actor) -> Integer to Bit Converter2/1
  Trigger/1 -> MATLAB Function1/Trigger
  MATLAB Function/1(signal) -> Send1/1

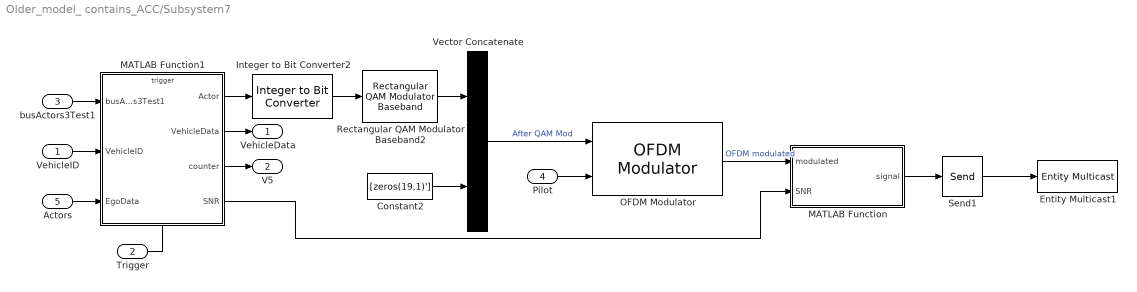
== system Older_model_ contains_ACC/Subsystem7 ==
  VehicleID : Inport
  Trigger : Inport  Port=2
  busActors3Test1 : Inport  Port=3
  Pilot : Inport  Port=4
  Actors : Inport  Port=5
  Constant2 : Constant  Value=[zeros(19,1)']  SampleTime=-1
  Entity Multicast1 : EntityMulticast  InputPortMessageModes=m
  Integer to Bit Converter2 : simulink/Logic and Bit Operations/Integer to Bit Converter  nbits=16  signedInputValues=Signed  bitOrder=MSB first  outDtype=boolean
  MATLAB Function : MATLAB Function  TreatAsAtomicUnit=on
  MATLAB Function1 : MATLAB Function  TreatAsAtomicUnit=on
  OFDM Modulator : commofdm/OFDM Modulator  StatePerturbationForJacobian=1.0e-05  FFTLength=64  NumGuardBandCarriers=[0;0]  InsertDCNull=on  PilotInputPort=on  PilotCarrierIndices=[12; 26; 40; 54]  CyclicPrefixLength=32  Windowing=off  WindowLength=16  OversamplingFactor=3  NumSymbols=1  NumTransmitAntennas=1  SimulateUsing=Interpreted execution
  Rectangular QAM Modulator Baseband2 : commdigbbndam3/Rectangular QAM Modulator Baseband  M=2^6  InType=Bit  Enc=Binary  Mapping=[0:15]  PowType=Average Power  MinDist=2  AvgPow=P_Signal  PeakPow=1  Ph=0  outDtype=double  outWordLen=16  outUDDataType=sfix(16)  outFracLenMode=Best precision  outFracLen=15  outDataTypeStr=double  outLastDataTypeStr=double
      settings: LibrarySourceBlock=|
      | commhdldigbbndam/Rectangular QAM
      | Modulator
      | Baseband
  Send1 : Send  OutputPortMessageModes=m
  Vector Concatenate : Concatenate
  VehicleData : Outport
  V5 : Outport  Port=2
  wires:
  MATLAB Function1/4(SNR) -> MATLAB Function/2(SNR)
  MATLAB Function1/3(counter) -> V5/1
  MATLAB Function1/2(VehicleData) -> VehicleData/1
  Pilot/1 -> OFDM Modulator/2
  VehicleID/1 -> MATLAB Function1/2(VehicleID)
  busActors3Test1/1 -> MATLAB Function1/1(busActors3Test1)
  Integer to Bit Converter2/1 -> Rectangular QAM Modulator Baseband2/1
  OFDM Modulator/1 -> MATLAB Function/1(modulated)  "OFDM modulated"
  Actors/1 -> MATLAB Function1/3(EgoData)
  Constant2/1 -> Vector Concatenate/2
  Rectangular QAM Modulator Baseband2/1 -> Vector Concatenate/1
  Send1/1 -> Entity Multicast1/1
  Vector Concatenate/1 -> OFDM Modulator/1  "After QAM Mod"
  MATLAB Function1/1(Actor) -> Integer to Bit Converter2/1
  Trigger/1 -> MATLAB Function1/Trigger
  MATLAB Function/1(signal) -> Send1/1

== system Older_model_ contains_ACC/Vehicle 2 ==
  trigger : Inport
  VehicleID : Inport  Port=2
  Pilot : Inport  Port=3
  busActors3Test1 : Inport  Port=4
  Constant2 : Constant  Value=[zeros(19,1)']  SampleTime=-1
  Entity Multicast1 : EntityMulticast  InputPortMessageModes=m
  Integer to Bit Converter1 : simulink/Logic and Bit Operations/Integer to Bit Converter  nbits=16  signedInputValues=Signed  bitOrder=MSB first  outDtype=boolean
  MATLAB Function1 : MATLAB Function  TreatAsAtomicUnit=on
  OFDM Modulator1 : commofdm/OFDM Modulator  StatePerturbationForJacobian=1.0e-05  FFTLength=64  NumGuardBandCarriers=[0;0]  InsertDCNull=on  PilotInputPort=on  PilotCarrierIndices=[12; 26; 40; 54]  CyclicPrefixLength=32  Windowing=off  WindowLength=16  OversamplingFactor=3  NumSymbols=1  NumTransmitAntennas=1  SimulateUsing=Interpreted execution
  Rectangular QAM Modulator Baseband1 : commdigbbndam3/Rectangular QAM Modulator Baseband  M=2^6  InType=Bit  Enc=Binary  Mapping=[0:15]  PowType=Average Power  MinDist=2  AvgPow=P_Signal  PeakPow=1  Ph=0  outDtype=double  outWordLen=16  outUDDataType=sfix(16)  outFracLenMode=Best precision  outFracLen=15  outDataTypeStr=double  outLastDataTypeStr=double
      settings: LibrarySourceBlock=|
      | commhdldigbbndam/Rectangular QAM
      | Modulator
      | Baseband
  Send1 : Send  OutputPortMessageModes=m
  Vector Concatenate1 : Concatenate
  wires:
  busActors3Test1/1 -> MATLAB Function1/1(busActors3Test1)
  Rectangular QAM Modulator Baseband1/1 -> Vector Concatenate1/1
  Constant2/1 -> Vector Concatenate1/2
  Send1/1 -> Entity Multicast1/1
  Integer to Bit Converter1/1 -> Rectangular QAM Modulator Baseband1/1
  Vector Concatenate1/1 -> OFDM Modulator1/1  "After QAM Mod"
  OFDM Modulator1/1 -> Send1/1  "OFDM modulated"
  MATLAB Function1/1(intVector) -> Integer to Bit Converter1/1
  trigger/1 -> MATLAB Function1/Trigger
  VehicleID/1 -> MATLAB Function1/2(VehicleID)
  Pilot/1 -> OFDM Modulator1/2

== system Older_model_ contains_ACC/Vehicle 3 ==
  trigger : Inport
  busActors3Test1 : Inport  Port=2
  Pilot : Inport  Port=3
  VehicleID : Inport  Port=4
  Constant3 : Constant  Value=[zeros(19,1)']  SampleTime=-1
  Entity Multicast2 : EntityMulticast  InputPortMessageModes=m
  Integer to Bit Converter3 : simulink/Logic and Bit Operations/Integer to Bit Converter  nbits=16  signedInputValues=Signed  bitOrder=MSB first  outDtype=boolean
  MATLAB Function2 : MATLAB Function  TreatAsAtomicUnit=on
  OFDM Modulator2 : commofdm/OFDM Modulator  StatePerturbationForJacobian=1.0e-05  FFTLength=64  NumGuardBandCarriers=[0;0]  InsertDCNull=on  PilotInputPort=on  PilotCarrierIndices=[12; 26; 40; 54]  CyclicPrefixLength=32  Windowing=off  WindowLength=16  OversamplingFactor=3  NumSymbols=1  NumTransmitAntennas=1  SimulateUsing=Interpreted execution
  Rectangular QAM Modulator Baseband3 : commdigbbndam3/Rectangular QAM Modulator Baseband  M=2^6  InType=Bit  Enc=Binary  Mapping=[0:15]  PowType=Average Power  MinDist=2  AvgPow=P_Signal  PeakPow=1  Ph=0  outDtype=double  outWordLen=16  outUDDataType=sfix(16)  outFracLenMode=Best precision  outFracLen=15  outDataTypeStr=double  outLastDataTypeStr=double
      settings: LibrarySourceBlock=|
      | commhdldigbbndam/Rectangular QAM
      | Modulator
      | Baseband
  Send2 : Send  OutputPortMessageModes=m
  Vector Concatenate2 : Concatenate
  wires:
  MATLAB Function2/1(intVector) -> Integer to Bit Converter3/1
  OFDM Modulator2/1 -> Send2/1  "OFDM modulated"
  busActors3Test1/1 -> MATLAB Function2/1(busActors3Test1)
  Vector Concatenate2/1 -> OFDM Modulator2/1  "After QAM Mod"
  Send2/1 -> Entity Multicast2/1
  Integer to Bit Converter3/1 -> Rectangular QAM Modulator Baseband3/1
  Rectangular QAM Modulator Baseband3/1 -> Vector Concatenate2/1
  Pilot/1 -> OFDM Modulator2/2
  Constant3/1 -> Vector Concatenate2/2
  VehicleID/1 -> MATLAB Function2/2(VehicleID)
  trigger/1 -> MATLAB Function2/Trigger

== system Older_model_ contains_ACC/channel ==
  Entity Multicast : EntityMulticast  InputPortMessageModes=m  MulticastTag=B
  MATLAB Function : MATLAB Function  Commented=through  TreatAsAtomicUnit=on
  Multicast Receive Queue : Queue  OutputPortMessageModes=m  EntityArrivalSource=Multicast
  Receive : Receive  InputPortMessageModes=m  UseInternalQueue=off  QueueOverwriting=on  QueueLength=1  QueueType=LIFO
  Send : Send  OutputPortMessageModes=m
  wires:
  Multicast Receive Queue/1 -> Receive/1
  Receive/1 -> MATLAB Function/1(u)
  MATLAB Function/1(y) -> Send/1
  Send/1 -> Entity Multicast/1

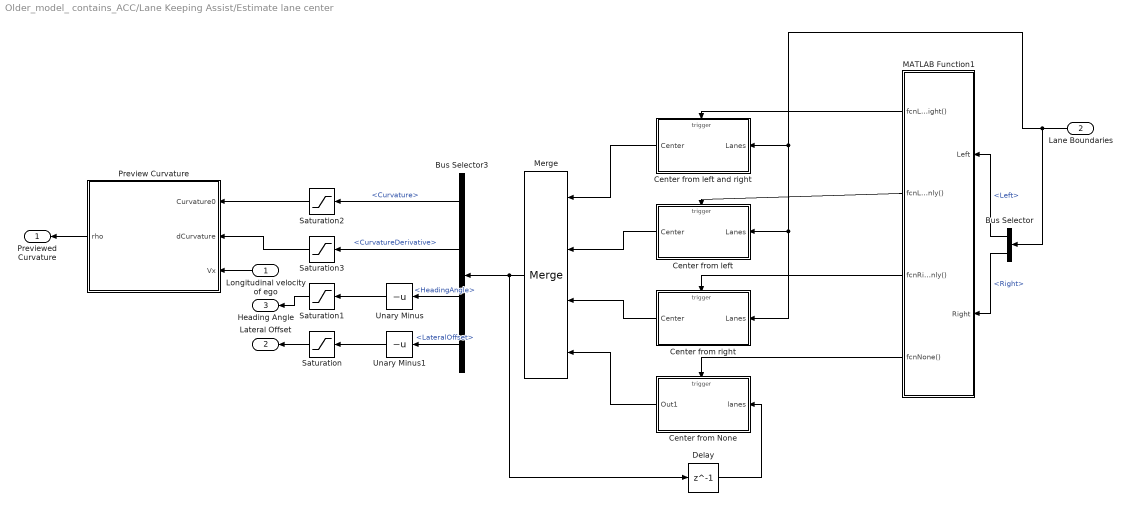
== system Older_model_ contains_ACC/Lane Keeping Assist/Estimate lane center ==
  Longitudinal velocity of ego : Inport
  Lane Boundaries : Inport  Port=2
  Bus Selector : BusSelector  OutputSignals=Left,Right
  Bus Selector3 : BusSelector  OutputSignals=Curvature,CurvatureDerivative,HeadingAngle,LateralOffset
  Center from None : Subsystem
  Center from left : Subsystem
  Center from left and right : Subsystem
  Center from right : Subsystem
  Delay : Delay  DelayLength=1
  MATLAB Function1 : MATLAB Function  TreatAsAtomicUnit=on
  Merge : Merge  Inputs=4  InputPortOffsets=4
  Preview Curvature : MATLAB Function  TreatAsAtomicUnit=on  SystemSampleTime=Ts
  Saturation : Saturate
  Saturation1 : Saturate  UpperLimit=0.6  LowerLimit=-0.6
  Saturation2 : Saturate  UpperLimit=0.15  LowerLimit=-0.15
  Saturation3 : Saturate  UpperLimit=0.06  LowerLimit=-0.06
  Unary Minus : UnaryMinus
  Unary Minus1 : UnaryMinus
  Previewed Curvature : Outport
  Lateral Offset : Outport  Port=2
  Heading Angle : Outport  Port=3
  wires:
  Bus Selector3/1 -> Saturation2/1  "<Curvature>"
  Bus Selector3/2 -> Saturation3/1  "<CurvatureDerivative>"
  Bus Selector3/4 -> Unary Minus1/1  "<LateralOffset>"
  Saturation1/1 -> Heading Angle/1
  Bus Selector3/3 -> Unary Minus/1  "<HeadingAngle>"
  MATLAB Function1/1(fcnLeftAndRight()) -> Center from left and right/Trigger
  MATLAB Function1/2(fcnLeftOnly()) -> Center from left/Trigger
  Saturation3/1 -> Preview Curvature/2(dCurvature)
  MATLAB Function1/3(fcnRightOnly()) -> Center from right/Trigger
  Unary Minus/1 -> Saturation1/1
  Delay/1 -> Center from None/1(lanes)
  MATLAB Function1/4(fcnNone()) -> Center from None/Trigger
  Saturation2/1 -> Preview Curvature/1(Curvature0)
  Unary Minus1/1 -> Saturation/1
  Preview Curvature/1(rho) -> Previewed Curvature/1
  Saturation/1 -> Lateral Offset/1
  Longitudinal velocity of ego/1 -> Preview Curvature/3(Vx)
  Lane Boundaries/1 -> Bus Selector/1, Center from left/1(Lanes), Center from right/1(Lanes), Center from left and right/1(Lanes)
  Bus Selector/1 -> MATLAB Function1/1(Left)  "<Left>"
  Bus Selector/2 -> MATLAB Function1/2(Right)  "<Right>"
  Center from None/1(Out1) -> Merge/4
  Center from left and right/1(Center) -> Merge/1
  Center from right/1(Center) -> Merge/3
  Center from left/1(Center) -> Merge/2
  Merge/1 -> Delay/1, Bus Selector3/1
